simulink model "MSDRPrimaryLoop"  (R2021b)
settings: Solver=VariableStepAuto  StartTime=0.0  StopTime=250000  MaxStep=1  MinStep=0.01  RelTol=1e-3
undefined symbols (not defined in the file): a_f, A_free_PHX, a_g, A_h_PHX, beta, beta_t, bubbleGeneratorArea, bubbleGeneratorDh, bubbleGeneratorElevation, bubbleGeneratorLength, bubbleGeneratorVolume, bubbleSaturationLevel, bubbleSeparatorArea, bubbleSeparatorDiameter, bubbleSeparatorDo, bubbleSeparatorLength, bubbleSeparatorSlope, bypassRatio, C0, coreFlowArea, coreFuelVolume, coreLowerPlenumArea, coreLowerPlenumHydraulicDiameter, coreLowerPlenumLength, coreLowerPlenumVolume, coreUpperPlenumArea, coreUpperPlenumHydraulicDiameter, coreUpperPlenumLength, coreUpperPlenumVolume, coreVolume, cpGraphite, dissolusionRatio, dMin, dScale, dsmConst, DXeG, Fiss_factor, fuelChannelHydrualicDiameter, fuelChannelLength, fuelDepositRatio, fuelFraction, fuelGraphiteArea, fuelGraphiteHeatTransferCoefficient, gamma0, gamma1, gamma2, generatorDsm, graphiteKDiff, graphiteUnitCellThickness, initialIodineConcentration, InitialXeMolarConcentration, InjectionRatio, injectionRatio, iodineDecayConstant, IodineDecayConstant, iodineYield, kGraphite, kScale, Lam, lam ... (+59)
libraries: fl_lib x272, nesl_utility x105, SimscapeFluids_lib x24, slpidlib x1
(part 2 of 12)

== system MSDRPrimaryLoop/Chemical Processing/Bubble Generator ==
  XeIn : Inport
  GasIn : Inport  Port=2
  Add : Sum  Inputs=|++
  Delay One Step : Delay  DelayLength=1
  Gain : Gain  Gain=0.5
  GasCalc : Subsystem  mask{Volume=bubbleGeneratorVolume, VoidFraction=targetGeneratorVoidFraction}
      mask prompts: VoidFraction "TargetVoidFraction"
      settings: PortSchema="{\"entries\":[{\"content\":{\"sides\":[{\"content\":{\"connectorIds\":[\"In1\"]},\"type\":\"ConnectorPlacement.EquallySpacedRectSide\",\"uuid\":\"a8e1ce06-71c9-462d-8d5c-7a3e078b5544\"},{\"content\":{\"connectorIds\":[\"Out1\"],\"side\":\"RIGHT\"},\"type\":\"ConnectorPlacement.EquallySpacedRectSide\",\"uuid\":\"2c63a1ce-15e2-4b17-a432-f9f40781bd58\"},{\"content\":{\"connectorIds\":[\"LConn1\",\"LConn2\",\"LConn3\"],\"side\":\"TOP\"},\"type\":\"ConnectorPlacement.EquallySpacedRectSide\",\"uuid\":\"abc20e07-15eb-475f-be7f-cc96378523a1\"},{\"content\":{\"connectorIds\":[],\"side\":\"BOTTOM\"},\"type\":\"ConnectorPlacement.EquallySpacedRectSide\",\"uuid\":\"ab58f362-f4c2-4e86-bda0-802426066295\"}]},\"type\":\"ConnectorPlacement.EquallySpacedConnector\",\"uuid\":\"b54d49a9-048b-4912-bf18-92a7ef5e8aff\"}],\"packageUris\":[\"http://schema.mathworks.com/mf0/Connector/R2020b\"],\"version\":\"1.0\"}"
  PLossFunc : Subsystem
      settings: PortSchema="{\"entries\":[{\"content\":{\"sides\":[{\"content\":{\"connectorIds\":[\"Out1\",\"LConn1\"]},\"type\":\"ConnectorPlacement.EquallySpacedRectSide\",\"uuid\":\"95ca4545-c473-4e31-844b-c43557042c16\"},{\"content\":{\"connectorIds\":[\"RConn1\"],\"side\":\"RIGHT\"},\"type\":\"ConnectorPlacement.EquallySpacedRectSide\",\"uuid\":\"f9304c30-8684-4a05-a34b-3121610e628d\"},{\"content\":{\"connectorIds\":[],\"side\":\"TOP\"},\"type\":\"ConnectorPlacement.EquallySpacedRectSide\",\"uuid\":\"64c7a4d8-8539-4303-ae81-4015bd1451af\"}]},\"type\":\"ConnectorPlacement.EquallySpacedConnector\",\"uuid\":\"40c12b2f-fb9d-4a19-b6f1-e93ae1fd4d68\"}],\"packageUris\":[\"http://schema.mathworks.com/mf0/Connector/R2020b\"],\"version\":\"1.0\"}"
  Subsystem : Subsystem  mask{Volume=bubbleGeneratorArea*bubbleGeneratorLength, Area=bubbleGeneratorArea, Length=bubbleGeneratorLength, Dh=bubbleGeneratorDh, Elevation=bubbleGeneratorElevation, MinimumArea=bubbleGeneratorArea*0.5}
      mask prompts: Dh "Hydraulic Diameter"; MinimumArea "VenturiMinimumArea"
      settings: PortSchema="{\"entries\":[{\"content\":{\"sides\":[{\"content\":{\"connectorIds\":[\"LConn1\",\"In1\"]},\"type\":\"ConnectorPlacement.EquallySpacedRectSide\",\"uuid\":\"0f255306-ec83-4423-ac41-a2708bd1ec44\"},{\"content\":{\"connectorIds\":[\"RConn1\"],\"side\":\"RIGHT\"},\"type\":\"ConnectorPlacement.EquallySpacedRectSide\",\"uuid\":\"650fb4ea-7b32-4c45-8538-9785d9ca64bf\"},{\"content\":{\"connectorIds\":[],\"side\":\"TOP\"},\"type\":\"ConnectorPlacement.EquallySpacedRectSide\",\"uuid\":\"434d3568-54a4-4787-a287-69f15ef478cb\"},{\"content\":{\"connectorIds\":[\"RConn2\"],\"side\":\"BOTTOM\"},\"type\":\"ConnectorPlacement.EquallySpacedRectSide\",\"uuid\":\"5b0b510d-1175-4508-bbe9-65b563e28484\"}]},\"type\":\"ConnectorPlacement.EquallySpacedConnector\",\"uuid\":\"b18d9c84-3d71-444b-a89d-79c3dc70d4d9\"}],\"packageUris\":[\"http://schema.mathworks.com/mf0/Connector/R2020b\"],\"version\":\"1.0\"}"
  XenonCalc : Subsystem  mask{Volume=bubbleGeneratorVolume, Area=bubbleGeneratorArea, Length=bubbleGeneratorLength, Dh=bubbleGeneratorDh, Elevation=bubbleGeneratorElevation, Dsm=generatorDsm}
      mask prompts: Dh "Hydraulic Diameter"; Dsm "InjectedBubbleDiameter"
      settings: PortSchema="{\"entries\":[{\"content\":{\"sides\":[{\"content\":{\"connectorIds\":[\"LConn1\",\"In1\"]},\"type\":\"ConnectorPlacement.EquallySpacedRectSide\",\"uuid\":\"82f8e7e7-fd89-4597-952e-64db268d0190\"},{\"content\":{\"connectorIds\":[\"RConn1\",\"Out1\"],\"side\":\"RIGHT\"},\"type\":\"ConnectorPlacement.EquallySpacedRectSide\",\"uuid\":\"4b3edad1-18f8-43fa-96ee-a24bb3384b59\"},{\"content\":{\"connectorIds\":[\"In2\"],\"side\":\"TOP\"},\"type\":\"ConnectorPlacement.EquallySpacedRectSide\",\"uuid\":\"43d4f51d-f841-40d6-804e-7f238a90dabe\"},{\"content\":{\"connectorIds\":[\"In3\"],\"side\":\"BOTTOM\"},\"type\":\"ConnectorPlacement.EquallySpacedRectSide\",\"uuid\":\"350f2274-4108-4e6e-a637-0ae7118de3f0\"}]},\"type\":\"ConnectorPlacement.EquallySpacedConnector\",\"uuid\":\"d7e795ea-9d5d-4a8c-83ab-dab42197cc2f\"}],\"packageUris\":[\"http://schema.mathworks.com/mf0/Connector/R2020b\"],\"version\":\"1.0\"}"
  Inlet : PMIOPort  Side=Left
  Outlet : PMIOPort  Port=2  Side=Right
  XeOut : Outport
  GasOut : Outport  Port=2
  wires:
  XenonCalc/1(XeOut) -> XeOut/1
  Add/1 -> Gain/1
  GasCalc/1(GasOut) -> GasOut/1, Add/2
  Gain/1 -> Delay One Step/1
  GasIn/1 -> GasCalc/1(GasIn), Add/1
  Delay One Step/1 -> XenonCalc/3(GasRef), Subsystem/1(GasInRef)
  XeIn/1 -> XenonCalc/1(XeIn)
  PLossFunc/1(PLoss) -> XenonCalc/2(PLoss)
  connections:
  GasCalc/LConn1 -- XenonCalc/LConn1 -- Inlet/RConn1
  GasCalc/LConn3 -- PLossFunc/RConn1 -- Outlet/RConn1 -- Subsystem/RConn1
  GasCalc/LConn2 -- Subsystem/RConn2
  PLossFunc/LConn1 -- XenonCalc/RConn1 -- Subsystem/LConn1

== system MSDRPrimaryLoop/Chemical Processing/Bubble Separator ==
  XeIn : Inport  OutDataTypeStr=double  Unit=kg/s
  GasIn : Inport  Port=2
  Constant : Constant
  Demux : Demux  Outputs=2
  Mux : Mux  Inputs=2
  PS Abs : fl_lib/Physical Signals/Nonlinear Operators/PS Abs
      settings: SourceProductBaseCode=SS  InternalSimscapePortConfiguration="{\"Bottom\":[],\"Left\":[{\"id\":\"I\",\"label\":\"\",\"type\":\"input\"}],\"Right\":[{\"id\":\"O\",\"label\":\"\",\"type\":\"output\"}],\"Top\":[]}"
  PS-Simulink Converter : nesl_utility/PS-Simulink Converter  PhysicalDomain=network_engine_domain  SubClassName=ps_output  LeftPortType=input  RightPortType=output  PseudoPeriodic=off  Frequencies=[]  Unit=inherit  AffineConversion=off
      settings: SourceProductBaseCode=PW,SS
  Pipe (TL) : SimscapeFluids_lib/Thermal Liquid/Pipes & Fittings/Pipe (TL)  dynamic_compressibility=simscape.enum.onoff.on  inertia=simscape.enum.onoff.off  num_segments=1  pipe_length=bubbleSeparatorLength m  area=bubbleSeparatorArea m^2  Dh=bubbleSeparatorDiameter m  wall_spec=fluids.thermal_liquid.pipes_fittings.enum.wall_spec.rigid  Dh_rigid=bubbleSeparatorDiameter m  wall_compliance=1.2e-6 m/MPa  wall_time_constant=0.01 s  elevation_spec=foundation.enum.constant_variable.constant  elevation_gain=0 m  g=9.81 m/s^2  pressure_loss_spec=fluids.thermal_liquid.pipes_fittings.enum.PressureLossSpec.Haaland  length_add=1 m  roughness=15e-6 m  Re_friction_TLU=[400, 1000, 1500, 3000, 4000, 6000, 10000, 20000, 40000, 60000, 100000, 100000000]  friction_factor_TLU=[.264, .112, .071, .0417, .0387, .0268, .025, .0232, .0226, .022, .0214, .0214]  shape_factor=64  Re_lam=2000  Re_tur=4000  mdot_nominal=[.1, 1] kg/s  p_diff_nominal=[.001, .01] MPa  mdot_threshold=1e-6 kg/s  heat_transfer_spec=fluids.thermal_liquid.pipes_fittings.enum.HeatTransferSpec.Gnielinski  mdot_nominal_heat=[.1, 1] kg/s  T_in_nominal=[293.15, 293.15] K  T_out_nominal=[300, 300] K  p_in_nominal_heat=[.101325, .101325] MPa  T_wall_nominal=[303.15, 303.15] K  a_coeff=0.023  b_Re_power=0.8  c_Pr_power=0.4  Nu_lam=3.66  Re_Colburn_TLU=[100, 150, 1000]  Colburn_factor_TLU=[.019, .013, .002]  Re_Nu_TLU=[100, 150, 1000]  Pr_Nu_TLU=[1, 10]  Nu_TLU=[3.72, 4.21; 3.75, 4.44; 4.21, 7.15]  T0_vec=T0 K  p0_vec=P0 Pa  mdot0=0.1 kg/s
      settings: SourceProductBaseCode=SH
  Product : Product
  Subsystem : Subsystem
      settings: PortSchema="{\"entries\":[{\"content\":{\"sides\":[{\"content\":{\"connectorIds\":[\"In1\",\"In2\"]},\"type\":\"ConnectorPlacement.EquallySpacedRectSide\",\"uuid\":\"428c9e87-9ca6-4187-8542-12893d09804c\"},{\"content\":{\"connectorIds\":[\"Out1\"],\"side\":\"RIGHT\"},\"type\":\"ConnectorPlacement.EquallySpacedRectSide\",\"uuid\":\"49ffe6be-5da6-43ae-9c06-12a699a32540\"},{\"content\":{\"connectorIds\":[\"Out2\"],\"side\":\"TOP\"},\"type\":\"ConnectorPlacement.EquallySpacedRectSide\",\"uuid\":\"09f5b805-0e4a-4494-a05c-730d3143cb28\"},{\"content\":{\"connectorIds\":[\"RConn1\"],\"side\":\"BOTTOM\"},\"type\":\"ConnectorPlacement.EquallySpacedRectSide\",\"uuid\":\"f4e426df-1694-4b1d-823a-475b1a6b135f\"}]},\"type\":\"ConnectorPlacement.EquallySpacedConnector\",\"uuid\":\"8fc0cfcf-d77b-45e0-be8a-b32970fc4d69\"}],\"packageUris\":[\"http://schema.mathworks.com/mf0/Connector/R2020b\"],\"version\":\"1.0\"}"
  Subtract : Sum  Inputs=+-
  To Workspace : ToWorkspace  VariableName=divertedFlowRate  SaveFormat=Timeseries  SampleTime=50
  To Workspace2 : ToWorkspace  VariableName=separatorEffList  SaveFormat=Timeseries  SampleTime=50
  Volumetric Flow Rate Sensor (TL) : fl_lib/Thermal Liquid/Sensors/Volumetric Flow Rate Sensor (TL)
      settings: SourceProductBaseCode=SS  InternalSimscapePortConfiguration="{\"Bottom\":[],\"Left\":[{\"id\":\"A\",\"label\":\"A\",\"type\":\"foundation.thermal_liquid.thermal_liquid\"}],\"Right\":[{\"id\":\"B\",\"label\":\"B\",\"type\":\"foundation.thermal_liquid.thermal_liquid\"},{\"id\":\"V\",\"label\":\"V\",\"type\":\"output\"}],\"Top\":[]}"
  Inlet : PMIOPort  Side=Left
  Outlet : PMIOPort  Port=2  Side=Right
  XeOut : Outport
  GasOut : Outport  Port=2
  wires:
  XeIn/1 -> Demux/1
  Mux/1 -> XeOut/1
  Demux/1 -> Mux/1
  GasIn/1 -> Subsystem/1(GasIn)
  Subsystem/1(GasOut) -> GasOut/1
  PS-Simulink Converter/1 -> To Workspace/1, Subsystem/2(volRate)
  Constant/1 -> Subtract/1
  Demux/2 -> Product/1
  Subtract/1 -> Product/2
  Product/1 -> Mux/2
  Subsystem/2(SepEff) -> To Workspace2/1, Subtract/2
  connections:
  Volumetric Flow Rate Sensor (TL)/RConn1 -- Subsystem/RConn1 -- Pipe (TL)/LConn1
  Volumetric Flow Rate Sensor (TL)/RConn2 -- PS Abs/LConn1
  PS-Simulink Converter/LConn1 -- PS Abs/RConn1
  Inlet/RConn1 -- Volumetric Flow Rate Sensor (TL)/LConn1
  Outlet/RConn1 -- Pipe (TL)/RConn1

== system MSDRPrimaryLoop/Chemical Processing/ElevationPipe ==
  XeIn : Inport
  GasIn : Inport  Port=2
  Add : Sum  Inputs=|++
  Delay One Step : Delay  DelayLength=1
  Gain : Gain  Gain=0.5
  GasCalc : Subsystem  mask{Volume=Volume}
      settings: PortSchema="{\"entries\":[{\"content\":{\"sides\":[{\"content\":{\"connectorIds\":[\"In1\"]},\"type\":\"ConnectorPlacement.EquallySpacedRectSide\",\"uuid\":\"a8e1ce06-71c9-462d-8d5c-7a3e078b5544\"},{\"content\":{\"connectorIds\":[\"Out1\"],\"side\":\"RIGHT\"},\"type\":\"ConnectorPlacement.EquallySpacedRectSide\",\"uuid\":\"2c63a1ce-15e2-4b17-a432-f9f40781bd58\"},{\"content\":{\"connectorIds\":[\"LConn1\",\"LConn2\",\"LConn3\"],\"side\":\"TOP\"},\"type\":\"ConnectorPlacement.EquallySpacedRectSide\",\"uuid\":\"abc20e07-15eb-475f-be7f-cc96378523a1\"},{\"content\":{\"connectorIds\":[],\"side\":\"BOTTOM\"},\"type\":\"ConnectorPlacement.EquallySpacedRectSide\",\"uuid\":\"ab58f362-f4c2-4e86-bda0-802426066295\"}]},\"type\":\"ConnectorPlacement.EquallySpacedConnector\",\"uuid\":\"b54d49a9-048b-4912-bf18-92a7ef5e8aff\"}],\"packageUris\":[\"http://schema.mathworks.com/mf0/Connector/R2020b\"],\"version\":\"1.0\"}"
  PLossFunc : Subsystem
      settings: PortSchema="{\"entries\":[{\"content\":{\"sides\":[{\"content\":{\"connectorIds\":[\"Out1\",\"LConn1\"]},\"type\":\"ConnectorPlacement.EquallySpacedRectSide\",\"uuid\":\"95ca4545-c473-4e31-844b-c43557042c16\"},{\"content\":{\"connectorIds\":[\"RConn1\"],\"side\":\"RIGHT\"},\"type\":\"ConnectorPlacement.EquallySpacedRectSide\",\"uuid\":\"f9304c30-8684-4a05-a34b-3121610e628d\"},{\"content\":{\"connectorIds\":[],\"side\":\"TOP\"},\"type\":\"ConnectorPlacement.EquallySpacedRectSide\",\"uuid\":\"64c7a4d8-8539-4303-ae81-4015bd1451af\"}]},\"type\":\"ConnectorPlacement.EquallySpacedConnector\",\"uuid\":\"40c12b2f-fb9d-4a19-b6f1-e93ae1fd4d68\"}],\"packageUris\":[\"http://schema.mathworks.com/mf0/Connector/R2020b\"],\"version\":\"1.0\"}"
  Subsystem : Subsystem  mask{Volume=Volume, Area=Area, Length=Length, Dh=Dh, Elevation=Elevation}
      mask prompts: Dh "Hydraulic Diameter"
      settings: PortSchema="{\"entries\":[{\"content\":{\"sides\":[{\"content\":{\"connectorIds\":[\"LConn1\",\"In1\"]},\"type\":\"ConnectorPlacement.EquallySpacedRectSide\",\"uuid\":\"0f255306-ec83-4423-ac41-a2708bd1ec44\"},{\"content\":{\"connectorIds\":[\"RConn1\"],\"side\":\"RIGHT\"},\"type\":\"ConnectorPlacement.EquallySpacedRectSide\",\"uuid\":\"650fb4ea-7b32-4c45-8538-9785d9ca64bf\"},{\"content\":{\"connectorIds\":[],\"side\":\"TOP\"},\"type\":\"ConnectorPlacement.EquallySpacedRectSide\",\"uuid\":\"434d3568-54a4-4787-a287-69f15ef478cb\"},{\"content\":{\"connectorIds\":[\"RConn2\"],\"side\":\"BOTTOM\"},\"type\":\"ConnectorPlacement.EquallySpacedRectSide\",\"uuid\":\"5b0b510d-1175-4508-bbe9-65b563e28484\"}]},\"type\":\"ConnectorPlacement.EquallySpacedConnector\",\"uuid\":\"b18d9c84-3d71-444b-a89d-79c3dc70d4d9\"}],\"packageUris\":[\"http://schema.mathworks.com/mf0/Connector/R2020b\"],\"version\":\"1.0\"}"
  XenonCalc : Subsystem  mask{Volume=Volume, Area=Area, Length=Length, Dh=Dh, Elevation=Elevation}
      mask prompts: Dh "Hydraulic Diameter"
      settings: PortSchema="{\"entries\":[{\"content\":{\"sides\":[{\"content\":{\"connectorIds\":[\"LConn1\",\"In1\"]},\"type\":\"ConnectorPlacement.EquallySpacedRectSide\",\"uuid\":\"82f8e7e7-fd89-4597-952e-64db268d0190\"},{\"content\":{\"connectorIds\":[\"RConn1\",\"Out1\"],\"side\":\"RIGHT\"},\"type\":\"ConnectorPlacement.EquallySpacedRectSide\",\"uuid\":\"4b3edad1-18f8-43fa-96ee-a24bb3384b59\"},{\"content\":{\"connectorIds\":[\"In2\"],\"side\":\"TOP\"},\"type\":\"ConnectorPlacement.EquallySpacedRectSide\",\"uuid\":\"43d4f51d-f841-40d6-804e-7f238a90dabe\"},{\"content\":{\"connectorIds\":[\"In3\"],\"side\":\"BOTTOM\"},\"type\":\"ConnectorPlacement.EquallySpacedRectSide\",\"uuid\":\"350f2274-4108-4e6e-a637-0ae7118de3f0\"}]},\"type\":\"ConnectorPlacement.EquallySpacedConnector\",\"uuid\":\"d7e795ea-9d5d-4a8c-83ab-dab42197cc2f\"}],\"packageUris\":[\"http://schema.mathworks.com/mf0/Connector/R2020b\"],\"version\":\"1.0\"}"
  Inlet : PMIOPort  Side=Left
  Outlet : PMIOPort  Port=2  Side=Right
  XeOut : Outport
  GasOut : Outport  Port=2
  wires:
  XenonCalc/1(XeOut) -> XeOut/1
  Add/1 -> Gain/1
  GasCalc/1(GasOut) -> GasOut/1, Add/2
  Gain/1 -> Delay One Step/1
  GasIn/1 -> GasCalc/1(GasIn), Add/1
  Delay One Step/1 -> XenonCalc/3(GasRef), Subsystem/1(GasInRef)
  XeIn/1 -> XenonCalc/1(XeIn)
  PLossFunc/1(PLoss) -> XenonCalc/2(PLoss)
  connections:
  GasCalc/LConn1 -- XenonCalc/LConn1 -- Inlet/RConn1
  GasCalc/LConn3 -- PLossFunc/RConn1 -- Outlet/RConn1 -- Subsystem/RConn1
  GasCalc/LConn2 -- Subsystem/RConn2
  PLossFunc/LConn1 -- XenonCalc/RConn1 -- Subsystem/LConn1

== system MSDRPrimaryLoop/Chemical Processing/PipeLine ==
  XeIn : Inport  OutDataTypeStr=double  Unit=kg/s
  GasIn : Inport  Port=2
  Add : Sum  Inputs=|++
  Delay One Step : Delay  DelayLength=1
  Gain : Gain  Gain=0.5
  GasCalc : Subsystem  mask{Volume=pipeLineVolume}
      settings: PortSchema="{\"entries\":[{\"content\":{\"sides\":[{\"content\":{\"connectorIds\":[\"In1\"]},\"type\":\"ConnectorPlacement.EquallySpacedRectSide\",\"uuid\":\"a8e1ce06-71c9-462d-8d5c-7a3e078b5544\"},{\"content\":{\"connectorIds\":[\"Out1\"],\"side\":\"RIGHT\"},\"type\":\"ConnectorPlacement.EquallySpacedRectSide\",\"uuid\":\"2c63a1ce-15e2-4b17-a432-f9f40781bd58\"},{\"content\":{\"connectorIds\":[\"LConn1\",\"LConn2\",\"LConn3\"],\"side\":\"TOP\"},\"type\":\"ConnectorPlacement.EquallySpacedRectSide\",\"uuid\":\"abc20e07-15eb-475f-be7f-cc96378523a1\"},{\"content\":{\"connectorIds\":[],\"side\":\"BOTTOM\"},\"type\":\"ConnectorPlacement.EquallySpacedRectSide\",\"uuid\":\"ab58f362-f4c2-4e86-bda0-802426066295\"}]},\"type\":\"ConnectorPlacement.EquallySpacedConnector\",\"uuid\":\"b54d49a9-048b-4912-bf18-92a7ef5e8aff\"}],\"packageUris\":[\"http://schema.mathworks.com/mf0/Connector/R2020b\"],\"version\":\"1.0\"}"
  PLossFunc : Subsystem
      settings: PortSchema="{\"entries\":[{\"content\":{\"sides\":[{\"content\":{\"connectorIds\":[\"Out1\",\"LConn1\"]},\"type\":\"ConnectorPlacement.EquallySpacedRectSide\",\"uuid\":\"95ca4545-c473-4e31-844b-c43557042c16\"},{\"content\":{\"connectorIds\":[\"RConn1\"],\"side\":\"RIGHT\"},\"type\":\"ConnectorPlacement.EquallySpacedRectSide\",\"uuid\":\"f9304c30-8684-4a05-a34b-3121610e628d\"},{\"content\":{\"connectorIds\":[],\"side\":\"TOP\"},\"type\":\"ConnectorPlacement.EquallySpacedRectSide\",\"uuid\":\"64c7a4d8-8539-4303-ae81-4015bd1451af\"}]},\"type\":\"ConnectorPlacement.EquallySpacedConnector\",\"uuid\":\"40c12b2f-fb9d-4a19-b6f1-e93ae1fd4d68\"}],\"packageUris\":[\"http://schema.mathworks.com/mf0/Connector/R2020b\"],\"version\":\"1.0\"}"
  Subsystem : Subsystem  mask{Volume=pipeLineVolume, Area=pipeLineArea, Length=pipeLineLength, Dh=pipeLineDh, Elevation=pipeLineElevation, KLoss=pipeLineKLoss}
      mask prompts: Dh "Hydraulic Diameter"; KLoss "TotalKLoss"
      settings: PortSchema="{\"entries\":[{\"content\":{\"sides\":[{\"content\":{\"connectorIds\":[\"LConn1\",\"In1\"]},\"type\":\"ConnectorPlacement.EquallySpacedRectSide\",\"uuid\":\"0f255306-ec83-4423-ac41-a2708bd1ec44\"},{\"content\":{\"connectorIds\":[\"RConn1\"],\"side\":\"RIGHT\"},\"type\":\"ConnectorPlacement.EquallySpacedRectSide\",\"uuid\":\"650fb4ea-7b32-4c45-8538-9785d9ca64bf\"},{\"content\":{\"connectorIds\":[],\"side\":\"TOP\"},\"type\":\"ConnectorPlacement.EquallySpacedRectSide\",\"uuid\":\"434d3568-54a4-4787-a287-69f15ef478cb\"},{\"content\":{\"connectorIds\":[\"RConn2\"],\"side\":\"BOTTOM\"},\"type\":\"ConnectorPlacement.EquallySpacedRectSide\",\"uuid\":\"5b0b510d-1175-4508-bbe9-65b563e28484\"}]},\"type\":\"ConnectorPlacement.EquallySpacedConnector\",\"uuid\":\"b18d9c84-3d71-444b-a89d-79c3dc70d4d9\"}],\"packageUris\":[\"http://schema.mathworks.com/mf0/Connector/R2020b\"],\"version\":\"1.0\"}"
  XenonCalc : Subsystem  mask{Volume=pipeLineVolume, Area=pipeLineArea, Length=pipeLineLength, Dh=pipeLineDh, Elevation=pipeLineElevation, Dsm=generatorDsm}
      mask prompts: Dh "Hydraulic Diameter"; Dsm "InjectedBubbleDiameter"
      settings: PortSchema="{\"entries\":[{\"content\":{\"sides\":[{\"content\":{\"connectorIds\":[\"LConn1\",\"In1\"]},\"type\":\"ConnectorPlacement.EquallySpacedRectSide\",\"uuid\":\"82f8e7e7-fd89-4597-952e-64db268d0190\"},{\"content\":{\"connectorIds\":[\"RConn1\",\"Out1\"],\"side\":\"RIGHT\"},\"type\":\"ConnectorPlacement.EquallySpacedRectSide\",\"uuid\":\"4b3edad1-18f8-43fa-96ee-a24bb3384b59\"},{\"content\":{\"connectorIds\":[\"In2\"],\"side\":\"TOP\"},\"type\":\"ConnectorPlacement.EquallySpacedRectSide\",\"uuid\":\"43d4f51d-f841-40d6-804e-7f238a90dabe\"},{\"content\":{\"connectorIds\":[\"In3\"],\"side\":\"BOTTOM\"},\"type\":\"ConnectorPlacement.EquallySpacedRectSide\",\"uuid\":\"350f2274-4108-4e6e-a637-0ae7118de3f0\"}]},\"type\":\"ConnectorPlacement.EquallySpacedConnector\",\"uuid\":\"d7e795ea-9d5d-4a8c-83ab-dab42197cc2f\"}],\"packageUris\":[\"http://schema.mathworks.com/mf0/Connector/R2020b\"],\"version\":\"1.0\"}"
  Inlet : PMIOPort  Side=Left
  Outlet : PMIOPort  Port=2  Side=Right
  XeOut : Outport
  GasOut : Outport  Port=2
  wires:
  PLossFunc/1(PLoss) -> XenonCalc/2(PLoss)
  XeIn/1 -> XenonCalc/1(XeIn)
  XenonCalc/1(XeOut) -> XeOut/1
  Gain/1 -> Delay One Step/1
  GasCalc/1(GasOut) -> GasOut/1, Add/2
  GasIn/1 -> GasCalc/1(GasIn), Add/1
  Add/1 -> Gain/1
  Delay One Step/1 -> XenonCalc/3(GasRef), Subsystem/1(GasInRef)
  connections:
  PLossFunc/RConn1 -- GasCalc/LConn3 -- Subsystem/RConn1 -- Outlet/RConn1
  GasCalc/LConn1 -- XenonCalc/LConn1 -- Inlet/RConn1
  XenonCalc/RConn1 -- Subsystem/LConn1 -- PLossFunc/LConn1
  GasCalc/LConn2 -- Subsystem/RConn2

== system MSDRPrimaryLoop/Chemical Processing/VariablePressureControl ==
  note: // This will be zero if not connected at both ends of the pump. Use physical connection first.
      | If no pump is used in the system, there has to be a pressure difference between the separator and the pump suction for the separator to work.
      | This could be think as a variable conection point on the primary loop. The Pressure drop here is summary of all the pressure loss after the varaible connection point.
  XeIn : Inport  OutDataTypeStr=double  Unit=kg/s
  GasIn : Inport  Port=2
  Flow Resistance (TL) : fl_lib/Thermal Liquid/Elements/Flow Resistance (TL)  delta_p_nominal=nominalSeparatorDP Pa  mdot_nominal=nominalSeparatorFlowRate*nominalFuelDensity kg/s  area=bubbleSeparatorArea m^2  laminar_fraction=1e-3
      settings: SourceProductBaseCode=SS
  GasExpansion : Subsystem  ReferencedSubsystem=GasExpansion
      settings: PortSchema="{\"entries\":[{\"content\":{\"sides\":[{\"content\":{\"connectorIds\":[\"LConn1\",\"In1\"]},\"type\":\"ConnectorPlacement.EquallySpacedRectSide\",\"uuid\":\"50c89675-cb8a-4964-af62-cb2014507b1d\"},{\"content\":{\"connectorIds\":[\"RConn1\",\"Out1\"],\"side\":\"RIGHT\"},\"type\":\"ConnectorPlacement.EquallySpacedRectSide\",\"uuid\":\"6b3adc78-0be5-4682-9da0-6fd41ffc4e71\"},{\"content\":{\"connectorIds\":[],\"side\":\"TOP\"},\"type\":\"ConnectorPlacement.EquallySpacedRectSide\",\"uuid\":\"5158b46f-a496-48e4-90d6-6c6dcc9e237b\"}]},\"type\":\"ConnectorPlacement.EquallySpacedConnector\",\"uuid\":\"7ff0188e-dc19-44a0-a8cf-bde33949414f\"}],\"packageUris\":[\"http://schema.mathworks.com/mf0/Connector/R2020b\"],\"version\":\"1.0\"}"
  Inlet : PMIOPort  Side=Left
  Outlet : PMIOPort  Port=2  Side=Right
  XeOut : Outport
  GasOut : Outport  Port=2
  wires:
  GasExpansion/1 -> GasOut/1
  GasIn/1 -> GasExpansion/1
  XeIn/1 -> XeOut/1
  connections:
  GasExpansion/RConn1 -- Outlet/RConn1 -- Flow Resistance (TL)/RConn1
  GasExpansion/LConn1 -- Inlet/RConn1 -- Flow Resistance (TL)/LConn1

== system MSDRPrimaryLoop/Converge/Mixing ==
  note: The gas stream can be easily handled with ratio of liquid phase.
  Xe1 : Inport
  Xe2 : Inport  Port=2
  Gas1 : Inport  Port=3
  Gas2 : Inport  Port=4
  Add : Sum
  Add1 : Sum
  PS-Simulink Converter : nesl_utility/PS-Simulink Converter  PhysicalDomain=network_engine_domain  SubClassName=ps_output  LeftPortType=input  RightPortType=output  PseudoPeriodic=off  Frequencies=[]  Unit=inherit  AffineConversion=off
      settings: SourceProductBaseCode=PW,SS
  PS-Simulink Converter1 : nesl_utility/PS-Simulink Converter  PhysicalDomain=network_engine_domain  SubClassName=ps_output  LeftPortType=input  RightPortType=output  PseudoPeriodic=off  Frequencies=[]  Unit=inherit  AffineConversion=off
      settings: SourceProductBaseCode=PW,SS
  Product : Product
  Product1 : Product
  Mix1 : PMIOPort  Side=Left
  Mix2 : PMIOPort  Port=2  Side=Left
  XeOut : Outport
  GasOut : Outport  Port=2
  wires:
  PS-Simulink Converter/1 -> Product1/2
  PS-Simulink Converter1/1 -> Product/2
  Gas2/1 -> Product/1
  Gas1/1 -> Product1/1
  Product1/1 -> Add/1
  Product/1 -> Add/2
  Add/1 -> GasOut/1
  Add1/1 -> XeOut/1
  Xe1/1 -> Add1/1
  Xe2/1 -> Add1/2
  connections:
  Mix1/RConn1 -- PS-Simulink Converter/LConn1
  Mix2/RConn1 -- PS-Simulink Converter1/LConn1

== system MSDRPrimaryLoop/Converge/PhysicalNetwork ==
  Mass & Energy Flow Rate Sensor (TL) : fl_lib/Thermal Liquid/Sensors/Mass & Energy Flow Rate Sensor (TL)
      settings: SourceProductBaseCode=SS  InternalSimscapePortConfiguration="{\"Bottom\":[],\"Left\":[{\"id\":\"A\",\"label\":\"A\",\"type\":\"foundation.thermal_liquid.thermal_liquid\"}],\"Right\":[{\"id\":\"B\",\"label\":\"B\",\"type\":\"foundation.thermal_liquid.thermal_liquid\"},{\"id\":\"M\",\"label\":\"M\",\"type\":\"output\"},{\"id\":\"PHI\",\"label\":\"Phi\",\"type\":\"output\"}],\"Top\":[]}"
  Mass & Energy Flow Rate Sensor (TL)1 : fl_lib/Thermal Liquid/Sensors/Mass & Energy Flow Rate Sensor (TL)
      settings: SourceProductBaseCode=SS  InternalSimscapePortConfiguration="{\"Bottom\":[],\"Left\":[{\"id\":\"A\",\"label\":\"A\",\"type\":\"foundation.thermal_liquid.thermal_liquid\"}],\"Right\":[{\"id\":\"B\",\"label\":\"B\",\"type\":\"foundation.thermal_liquid.thermal_liquid\"},{\"id\":\"M\",\"label\":\"M\",\"type\":\"output\"},{\"id\":\"PHI\",\"label\":\"Phi\",\"type\":\"output\"}],\"Top\":[]}"
  Mass & Energy Flow Rate Sensor (TL)2 : fl_lib/Thermal Liquid/Sensors/Mass & Energy Flow Rate Sensor (TL)
      settings: SourceProductBaseCode=SS  InternalSimscapePortConfiguration="{\"Bottom\":[],\"Left\":[{\"id\":\"A\",\"label\":\"A\",\"type\":\"foundation.thermal_liquid.thermal_liquid\"}],\"Right\":[{\"id\":\"B\",\"label\":\"B\",\"type\":\"foundation.thermal_liquid.thermal_liquid\"},{\"id\":\"M\",\"label\":\"M\",\"type\":\"output\"},{\"id\":\"PHI\",\"label\":\"Phi\",\"type\":\"output\"}],\"Top\":[]}"
  PS Abs : fl_lib/Physical Signals/Nonlinear Operators/PS Abs
      settings: SourceProductBaseCode=SS  InternalSimscapePortConfiguration="{\"Bottom\":[],\"Left\":[{\"id\":\"I\",\"label\":\"\",\"type\":\"input\"}],\"Right\":[{\"id\":\"O\",\"label\":\"\",\"type\":\"output\"}],\"Top\":[]}"
  PS Abs1 : fl_lib/Physical Signals/Nonlinear Operators/PS Abs
      settings: SourceProductBaseCode=SS  InternalSimscapePortConfiguration="{\"Bottom\":[],\"Left\":[{\"id\":\"I\",\"label\":\"\",\"type\":\"input\"}],\"Right\":[{\"id\":\"O\",\"label\":\"\",\"type\":\"output\"}],\"Top\":[]}"
  PS Abs2 : fl_lib/Physical Signals/Nonlinear Operators/PS Abs
      settings: SourceProductBaseCode=SS  InternalSimscapePortConfiguration="{\"Bottom\":[],\"Left\":[{\"id\":\"I\",\"label\":\"\",\"type\":\"input\"}],\"Right\":[{\"id\":\"O\",\"label\":\"\",\"type\":\"output\"}],\"Top\":[]}"
  PS Constant : fl_lib/Physical Signals/Sources/PS Constant  constant=1e-6 kg/s
  PS Divide : fl_lib/Physical Signals/Functions/PS Divide
      settings: SourceProductBaseCode=SS
  PS Divide1 : fl_lib/Physical Signals/Functions/PS Divide
      settings: SourceProductBaseCode=SS
  PS Max : fl_lib/Physical Signals/Nonlinear Operators/PS Max
      settings: SourceProductBaseCode=SS  InternalSimscapePortConfiguration="{\"Bottom\":[],\"Left\":[{\"id\":\"I1\",\"label\":\"\",\"type\":\"input\"},{\"id\":\"I2\",\"label\":\"\",\"type\":\"input\"}],\"Right\":[{\"id\":\"O\",\"label\":\"\",\"type\":\"output\"}],\"Top\":[]}"
  Subsystem : Subsystem
  MainIn : PMIOPort  Side=Left
  SideIn : PMIOPort  Port=2  Side=Left
  MainRatio : PMIOPort  Port=3  Side=Right
  SideRatio : PMIOPort  Port=4  Side=Right
  TotalOut : PMIOPort  Port=5  Side=Right
  connections:
  Subsystem/LConn1 -- Mass & Energy Flow Rate Sensor (TL)/RConn1
  Mass & Energy Flow Rate Sensor (TL)/RConn2 -- PS Abs/LConn1
  Mass & Energy Flow Rate Sensor (TL)/LConn1 -- MainIn/RConn1
  Subsystem/LConn2 -- Mass & Energy Flow Rate Sensor (TL)1/RConn1
  Mass & Energy Flow Rate Sensor (TL)1/RConn2 -- PS Abs1/LConn1
  Mass & Energy Flow Rate Sensor (TL)1/LConn1 -- SideIn/RConn1
  Subsystem/RConn1 -- Mass & Energy Flow Rate Sensor (TL)2/LConn1
  TotalOut/RConn1 -- Mass & Energy Flow Rate Sensor (TL)2/RConn1
  Mass & Energy Flow Rate Sensor (TL)2/RConn2 -- PS Abs2/LConn1
  PS Abs2/RConn1 -- PS Max/LConn1
  PS Max/LConn2 -- PS Constant/RConn1
  PS Abs1/RConn1 -- PS Divide/LConn1
  PS Max/RConn1 -- PS Divide1/LConn2 -- PS Divide/LConn2
  PS Divide/RConn1 -- SideRatio/RConn1
  PS Abs/RConn1 -- PS Divide1/LConn1
  PS Divide1/RConn1 -- MainRatio/RConn1

== system MSDRPrimaryLoop/Diverge/Subsystem1 ==
  note: Handle divide by zero.
  MainXeRate : fl_lib/Physical Signals/Functions/PS Divide
      settings: SourceProductBaseCode=SS
  Mass & Energy Flow Rate Sensor (TL) : fl_lib/Thermal Liquid/Sensors/Mass & Energy Flow Rate Sensor (TL)
      settings: SourceProductBaseCode=SS  InternalSimscapePortConfiguration="{\"Bottom\":[],\"Left\":[{\"id\":\"A\",\"label\":\"A\",\"type\":\"foundation.thermal_liquid.thermal_liquid\"}],\"Right\":[{\"id\":\"B\",\"label\":\"B\",\"type\":\"foundation.thermal_liquid.thermal_liquid\"},{\"id\":\"M\",\"label\":\"M\",\"type\":\"output\"},{\"id\":\"PHI\",\"label\":\"Phi\",\"type\":\"output\"}],\"Top\":[]}"
  Mass & Energy Flow Rate Sensor (TL)1 : fl_lib/Thermal Liquid/Sensors/Mass & Energy Flow Rate Sensor (TL)
      settings: SourceProductBaseCode=SS  InternalSimscapePortConfiguration="{\"Bottom\":[],\"Left\":[{\"id\":\"A\",\"label\":\"A\",\"type\":\"foundation.thermal_liquid.thermal_liquid\"}],\"Right\":[{\"id\":\"B\",\"label\":\"B\",\"type\":\"foundation.thermal_liquid.thermal_liquid\"},{\"id\":\"M\",\"label\":\"M\",\"type\":\"output\"},{\"id\":\"PHI\",\"label\":\"Phi\",\"type\":\"output\"}],\"Top\":[]}"
  Mass & Energy Flow Rate Sensor (TL)2 : fl_lib/Thermal Liquid/Sensors/Mass & Energy Flow Rate Sensor (TL)
      settings: SourceProductBaseCode=SS  InternalSimscapePortConfiguration="{\"Bottom\":[],\"Left\":[{\"id\":\"A\",\"label\":\"A\",\"type\":\"foundation.thermal_liquid.thermal_liquid\"}],\"Right\":[{\"id\":\"B\",\"label\":\"B\",\"type\":\"foundation.thermal_liquid.thermal_liquid\"},{\"id\":\"M\",\"label\":\"M\",\"type\":\"output\"},{\"id\":\"PHI\",\"label\":\"Phi\",\"type\":\"output\"}],\"Top\":[]}"
  PS Abs : fl_lib/Physical Signals/Nonlinear Operators/PS Abs
      settings: SourceProductBaseCode=SS  InternalSimscapePortConfiguration="{\"Bottom\":[],\"Left\":[{\"id\":\"I\",\"label\":\"\",\"type\":\"input\"}],\"Right\":[{\"id\":\"O\",\"label\":\"\",\"type\":\"output\"}],\"Top\":[]}"
  PS Abs1 : fl_lib/Physical Signals/Nonlinear Operators/PS Abs
      settings: SourceProductBaseCode=SS  InternalSimscapePortConfiguration="{\"Bottom\":[],\"Left\":[{\"id\":\"I\",\"label\":\"\",\"type\":\"input\"}],\"Right\":[{\"id\":\"O\",\"label\":\"\",\"type\":\"output\"}],\"Top\":[]}"
  PS Abs2 : fl_lib/Physical Signals/Nonlinear Operators/PS Abs
      settings: SourceProductBaseCode=SS  InternalSimscapePortConfiguration="{\"Bottom\":[],\"Left\":[{\"id\":\"I\",\"label\":\"\",\"type\":\"input\"}],\"Right\":[{\"id\":\"O\",\"label\":\"\",\"type\":\"output\"}],\"Top\":[]}"
  PS Constant : fl_lib/Physical Signals/Sources/PS Constant  constant=1e-6 kg/s
  PS Max : fl_lib/Physical Signals/Nonlinear Operators/PS Max
      settings: SourceProductBaseCode=SS  InternalSimscapePortConfiguration="{\"Bottom\":[],\"Left\":[{\"id\":\"I1\",\"label\":\"\",\"type\":\"input\"},{\"id\":\"I2\",\"label\":\"\",\"type\":\"input\"}],\"Right\":[{\"id\":\"O\",\"label\":\"\",\"type\":\"output\"}],\"Top\":[]}"
  PS-Simulink Converter : nesl_utility/PS-Simulink Converter  PhysicalDomain=network_engine_domain  SubClassName=ps_output  LeftPortType=input  RightPortType=output  PseudoPeriodic=off  Frequencies=[]  Unit=inherit  AffineConversion=off
      settings: SourceProductBaseCode=PW,SS
  PS-Simulink Converter2 : nesl_utility/PS-Simulink Converter  PhysicalDomain=network_engine_domain  SubClassName=ps_output  LeftPortType=input  RightPortType=output  PseudoPeriodic=off  Frequencies=[]  Unit=inherit  AffineConversion=off
      settings: SourceProductBaseCode=PW,SS
  SideXeRate : fl_lib/Physical Signals/Functions/PS Divide
      settings: SourceProductBaseCode=SS
  Subsystem : Subsystem
  Inlet : PMIOPort  Side=Left
  MainOut : PMIOPort  Port=2  Side=Right
  SideOut : PMIOPort  Port=3  Side=Right
  MainRatio : Outport
  SideRatio : Outport  Port=2
  wires:
  PS-Simulink Converter2/1 -> MainRatio/1
  PS-Simulink Converter/1 -> SideRatio/1
  connections:
  MainXeRate/LConn1 -- PS Abs2/RConn1
  Mass & Energy Flow Rate Sensor (TL)/RConn1 -- Subsystem/LConn1
  Mass & Energy Flow Rate Sensor (TL)1/RConn1 -- SideOut/RConn1
  Mass & Energy Flow Rate Sensor (TL)1/RConn2 -- PS Abs1/LConn1
  Mass & Energy Flow Rate Sensor (TL)1/LConn1 -- Subsystem/RConn2
  PS Abs/RConn1 -- PS Max/LConn1
  PS Constant/RConn1 -- PS Max/LConn2
  PS Abs1/RConn1 -- SideXeRate/LConn1
  MainXeRate/RConn1 -- PS-Simulink Converter2/LConn1
  PS Abs2/LConn1 -- Mass & Energy Flow Rate Sensor (TL)2/RConn2
  SideXeRate/RConn1 -- PS-Simulink Converter/LConn1
  PS Max/RConn1 -- MainXeRate/LConn2 -- SideXeRate/LConn2
  Mass & Energy Flow Rate Sensor (TL)/RConn2 -- PS Abs/LConn1
  Mass & Energy Flow Rate Sensor (TL)2/LConn1 -- Subsystem/RConn1
  Mass & Energy Flow Rate Sensor (TL)/LConn1 -- Inlet/RConn1
  Mass & Energy Flow Rate Sensor (TL)2/RConn1 -- MainOut/RConn1

== system MSDRPrimaryLoop/Ideal Expansion//Drain Tank/Coupled ==
  DrainTank : fl_lib/Thermal Liquid/Elements/Reservoir (TL)  pressure_spec=foundation.enum.pressure_spec.specified  reservoir_pressure=P0 Pa  reservoir_temperature=T0 K  area=0.01 m^2
      settings: SourceProductBaseCode=SS
  TotalIn : PMIOPort  Side=Left
  Inlet : PMIOPort  Port=2  Side=Right
  connections:
  Inlet/RConn1 -- TotalIn/RConn1 -- DrainTank/LConn1

== system MSDRPrimaryLoop/Ideal Expansion//Drain Tank/Segregate ==
  SimpleOverFlowTank : fl_lib/Thermal Liquid/Elements/Reservoir (TL)  pressure_spec=foundation.enum.pressure_spec.specified  reservoir_pressure=P0 Pa  reservoir_temperature=T0 K  area=0.01 m^2
      settings: SourceProductBaseCode=SS
  SimpleOverFlowTank1 : fl_lib/Thermal Liquid/Elements/Reservoir (TL)  pressure_spec=foundation.enum.pressure_spec.specified  reservoir_pressure=P0 Pa  reservoir_temperature=T0 K  area=0.01 m^2
      settings: SourceProductBaseCode=SS
  TotalIn : PMIOPort  Side=Left
  Inlet : PMIOPort  Port=2  Side=Right
  connections:
  SimpleOverFlowTank/LConn1 -- TotalIn/RConn1
  SimpleOverFlowTank1/LConn1 -- Inlet/RConn1

== system MSDRPrimaryLoop/PHX/PHX Ideal ==
  note: The outlet temperature of the PHX is controlled as a constant. The pressure drop is scaled with the square of the volume flowrate. This is primarily used for xenon calculation.
  XeIn : Inport
  GasIn : Inport  Port=2
  Add : Sum  Inputs=|++
  Delay One Step : Delay  DelayLength=1  InitialCondition=0.02
  Gain : Gain  Gain=0.5
  GasCalc : Subsystem  mask{PipeVolume=PHXVolume}
      mask prompts: PipeVolume "Volume"
      settings: PortSchema="{\"entries\":[{\"content\":{\"sides\":[{\"content\":{\"connectorIds\":[\"In1\"]},\"type\":\"ConnectorPlacement.EquallySpacedRectSide\",\"uuid\":\"a8e1ce06-71c9-462d-8d5c-7a3e078b5544\"},{\"content\":{\"connectorIds\":[\"Out1\"],\"side\":\"RIGHT\"},\"type\":\"ConnectorPlacement.EquallySpacedRectSide\",\"uuid\":\"2c63a1ce-15e2-4b17-a432-f9f40781bd58\"},{\"content\":{\"connectorIds\":[\"LConn1\",\"LConn2\",\"LConn3\"],\"side\":\"TOP\"},\"type\":\"ConnectorPlacement.EquallySpacedRectSide\",\"uuid\":\"abc20e07-15eb-475f-be7f-cc96378523a1\"},{\"content\":{\"connectorIds\":[],\"side\":\"BOTTOM\"},\"type\":\"ConnectorPlacement.EquallySpacedRectSide\",\"uuid\":\"ab58f362-f4c2-4e86-bda0-802426066295\"}]},\"type\":\"ConnectorPlacement.EquallySpacedConnector\",\"uuid\":\"b54d49a9-048b-4912-bf18-92a7ef5e8aff\"}],\"packageUris\":[\"http://schema.mathworks.com/mf0/Connector/R2020b\"],\"version\":\"1.0\"}"
  PHXIdeal : Subsystem
      settings: PortSchema="{\"entries\":[{\"content\":{\"sides\":[{\"content\":{\"connectorIds\":[\"LConn1\"]},\"type\":\"ConnectorPlacement.EquallySpacedRectSide\",\"uuid\":\"f66bece2-fdc4-4c5c-8b9b-b9978f494d53\"},{\"content\":{\"connectorIds\":[\"RConn1\"],\"side\":\"RIGHT\"},\"type\":\"ConnectorPlacement.EquallySpacedRectSide\",\"uuid\":\"48186cbd-a433-437a-a956-52e0dc00c30c\"},{\"content\":{\"connectorIds\":[],\"side\":\"TOP\"},\"type\":\"ConnectorPlacement.EquallySpacedRectSide\",\"uuid\":\"cd990d09-c0f9-4846-88b8-fe01d85fbb00\"},{\"content\":{\"connectorIds\":[\"RConn2\"],\"side\":\"BOTTOM\"},\"type\":\"ConnectorPlacement.EquallySpacedRectSide\",\"uuid\":\"c2d21c1c-5d2e-4128-be09-2d665ea38132\"}]},\"type\":\"ConnectorPlacement.EquallySpacedConnector\",\"uuid\":\"00e4a5dc-c184-4d43-a987-caabcada1902\"}],\"packageUris\":[\"http://schema.mathworks.com/mf0/Connector/R2020b\"],\"version\":\"1.0\"}"
  PS-Simulink Converter : nesl_utility/PS-Simulink Converter  PhysicalDomain=network_engine_domain  SubClassName=ps_output  LeftPortType=input  RightPortType=output  PseudoPeriodic=off  Frequencies=[]  Unit=inherit  AffineConversion=off
      settings: SourceProductBaseCode=PW,SS
  Pressure & Temperature Sensor (TL) : fl_lib/Thermal Liquid/Sensors/Pressure & Temperature Sensor (TL)
      settings: SourceProductBaseCode=SS  InternalSimscapePortConfiguration="{\"Bottom\":[],\"Left\":[{\"id\":\"A\",\"label\":\"A\",\"type\":\"foundation.thermal_liquid.thermal_liquid\"}],\"Right\":[{\"id\":\"B\",\"label\":\"B\",\"type\":\"foundation.thermal_liquid.thermal_liquid\"},{\"id\":\"P\",\"label\":\"P\",\"type\":\"output\"},{\"id\":\"T\",\"label\":\"T\",\"type\":\"output\"}],\"Top\":[]}"
  XenonCalc : Subsystem  mask{Volume=PHXVolume, Area=FlowArea, Length=PHXLength, Dh=PHXHydraulicDiameter, Elevation=0}
      mask prompts: Dh "Hydraulic Diameter"
      settings: PortSchema="{\"entries\":[{\"content\":{\"sides\":[{\"content\":{\"connectorIds\":[\"LConn1\",\"In1\"]},\"type\":\"ConnectorPlacement.EquallySpacedRectSide\",\"uuid\":\"82f8e7e7-fd89-4597-952e-64db268d0190\"},{\"content\":{\"connectorIds\":[\"RConn1\",\"Out1\"],\"side\":\"RIGHT\"},\"type\":\"ConnectorPlacement.EquallySpacedRectSide\",\"uuid\":\"4b3edad1-18f8-43fa-96ee-a24bb3384b59\"},{\"content\":{\"connectorIds\":[\"In2\"],\"side\":\"TOP\"},\"type\":\"ConnectorPlacement.EquallySpacedRectSide\",\"uuid\":\"43d4f51d-f841-40d6-804e-7f238a90dabe\"},{\"content\":{\"connectorIds\":[\"In3\"],\"side\":\"BOTTOM\"},\"type\":\"ConnectorPlacement.EquallySpacedRectSide\",\"uuid\":\"350f2274-4108-4e6e-a637-0ae7118de3f0\"}]},\"type\":\"ConnectorPlacement.EquallySpacedConnector\",\"uuid\":\"d7e795ea-9d5d-4a8c-83ab-dab42197cc2f\"}],\"packageUris\":[\"http://schema.mathworks.com/mf0/Connector/R2020b\"],\"version\":\"1.0\"}"
  Inlet : PMIOPort  Side=Left
  Outlet : PMIOPort  Port=2  Side=Right
  XeOut : Outport
  GasOut : Outport  Port=2
  wires:
  XenonCalc/1(XeOut) -> XeOut/1
  XeIn/1 -> XenonCalc/1(XeIn)
  Gain/1 -> Delay One Step/1
  Delay One Step/1 -> XenonCalc/3(GasRef)
  GasIn/1 -> GasCalc/1(GasIn), Add/1
  GasCalc/1(GasOut) -> GasOut/1, Add/2
  Add/1 -> Gain/1
  PS-Simulink Converter/1 -> XenonCalc/2(PLoss)
  connections:
  GasCalc/LConn2 -- PHXIdeal/RConn2
  PHXIdeal/RConn1 -- Pressure & Temperature Sensor (TL)/RConn1 -- Outlet/RConn1 -- GasCalc/LConn3
  PHXIdeal/LConn1 -- Pressure & Temperature Sensor (TL)/LConn1 -- XenonCalc/RConn1 -- GasCalc/LConn1
  XenonCalc/LConn1 -- Inlet/RConn1
  PS-Simulink Converter/LConn1 -- Pressure & Temperature Sensor (TL)/RConn2

== system MSDRPrimaryLoop/PHX/PHX Physical ==
  XeIn : Inport
  GasIn : Inport  Port=2
  Add : Sum  Inputs=|++
  Delay One Step : Delay  DelayLength=1
  Gain : Gain  Gain=0.5
  GasCalc1 : Subsystem  mask{PipeVolume=PHXVolume}
      mask prompts: PipeVolume "Volume"
      settings: PortSchema="{\"entries\":[{\"content\":{\"sides\":[{\"content\":{\"connectorIds\":[\"In1\"]},\"type\":\"ConnectorPlacement.EquallySpacedRectSide\",\"uuid\":\"a8e1ce06-71c9-462d-8d5c-7a3e078b5544\"},{\"content\":{\"connectorIds\":[\"Out1\"],\"side\":\"RIGHT\"},\"type\":\"ConnectorPlacement.EquallySpacedRectSide\",\"uuid\":\"2c63a1ce-15e2-4b17-a432-f9f40781bd58\"},{\"content\":{\"connectorIds\":[\"LConn1\",\"LConn2\",\"LConn3\"],\"side\":\"TOP\"},\"type\":\"ConnectorPlacement.EquallySpacedRectSide\",\"uuid\":\"abc20e07-15eb-475f-be7f-cc96378523a1\"},{\"content\":{\"connectorIds\":[],\"side\":\"BOTTOM\"},\"type\":\"ConnectorPlacement.EquallySpacedRectSide\",\"uuid\":\"ab58f362-f4c2-4e86-bda0-802426066295\"}]},\"type\":\"ConnectorPlacement.EquallySpacedConnector\",\"uuid\":\"b54d49a9-048b-4912-bf18-92a7ef5e8aff\"}],\"packageUris\":[\"http://schema.mathworks.com/mf0/Connector/R2020b\"],\"version\":\"1.0\"}"
  PHXPhysics : Subsystem
      settings: PortSchema="{\"entries\":[{\"content\":{\"sides\":[{\"content\":{\"connectorIds\":[\"LConn1\",\"In1\"]},\"type\":\"ConnectorPlacement.EquallySpacedRectSide\",\"uuid\":\"f66bece2-fdc4-4c5c-8b9b-b9978f494d53\"},{\"content\":{\"connectorIds\":[\"RConn1\"],\"side\":\"RIGHT\"},\"type\":\"ConnectorPlacement.EquallySpacedRectSide\",\"uuid\":\"48186cbd-a433-437a-a956-52e0dc00c30c\"},{\"content\":{\"connectorIds\":[],\"side\":\"TOP\"},\"type\":\"ConnectorPlacement.EquallySpacedRectSide\",\"uuid\":\"cd990d09-c0f9-4846-88b8-fe01d85fbb00\"},{\"content\":{\"connectorIds\":[\"RConn2\"],\"side\":\"BOTTOM\"},\"type\":\"ConnectorPlacement.EquallySpacedRectSide\",\"uuid\":\"c2d21c1c-5d2e-4128-be09-2d665ea38132\"}]},\"type\":\"ConnectorPlacement.EquallySpacedConnector\",\"uuid\":\"00e4a5dc-c184-4d43-a987-caabcada1902\"}],\"packageUris\":[\"http://schema.mathworks.com/mf0/Connector/R2020b\"],\"version\":\"1.0\"}"
  XenonCalc1 : Subsystem  mask{PipeVolume=PHXVolume, PipeArea=FlowArea, PipeLength=ChannelLength, Dh=Dh}
      mask prompts: PipeVolume "Volume"; PipeArea "Area"; PipeLength "Length"; Dh "Hydraulic Diameter"
      settings: PortSchema="{\"entries\":[{\"content\":{\"sides\":[{\"content\":{\"connectorIds\":[\"LConn1\",\"In1\"]},\"type\":\"ConnectorPlacement.EquallySpacedRectSide\",\"uuid\":\"82f8e7e7-fd89-4597-952e-64db268d0190\"},{\"content\":{\"connectorIds\":[\"RConn1\",\"Out1\"],\"side\":\"RIGHT\"},\"type\":\"ConnectorPlacement.EquallySpacedRectSide\",\"uuid\":\"4b3edad1-18f8-43fa-96ee-a24bb3384b59\"},{\"content\":{\"connectorIds\":[],\"side\":\"TOP\"},\"type\":\"ConnectorPlacement.EquallySpacedRectSide\",\"uuid\":\"43d4f51d-f841-40d6-804e-7f238a90dabe\"},{\"content\":{\"connectorIds\":[\"In2\"],\"side\":\"BOTTOM\"},\"type\":\"ConnectorPlacement.EquallySpacedRectSide\",\"uuid\":\"350f2274-4108-4e6e-a637-0ae7118de3f0\"}]},\"type\":\"ConnectorPlacement.EquallySpacedConnector\",\"uuid\":\"d7e795ea-9d5d-4a8c-83ab-dab42197cc2f\"}],\"packageUris\":[\"http://schema.mathworks.com/mf0/Connector/R2020b\"],\"version\":\"1.0\"}"
  Inlet : PMIOPort  Side=Left
  Outlet : PMIOPort  Port=2  Side=Right
  XeOut : Outport
  GasOut : Outport  Port=2
  wires:
  XenonCalc1/1(XeOut) -> XeOut/1
  XeIn/1 -> XenonCalc1/1(XeIn)
  Gain/1 -> Delay One Step/1
  Delay One Step/1 -> XenonCalc1/2(GasRef), PHXPhysics/1(GasInRef)
  GasIn/1 -> GasCalc1/1(GasIn), Add/1
  GasCalc1/1(GasOut) -> GasOut/1, Add/2
  Add/1 -> Gain/1
  connections:
  GasCalc1/LConn2 -- PHXPhysics/RConn2
  PHXPhysics/RConn1 -- Outlet/RConn1 -- GasCalc1/LConn3
  PHXPhysics/LConn1 -- GasCalc1/LConn1 -- XenonCalc1/RConn1
  XenonCalc1/LConn1 -- Inlet/RConn1

== system MSDRPrimaryLoop/Pump/PumpIdeal ==
  XeIn : Inport
  GasIn : Inport  Port=2
  Add : Sum  Inputs=|++
  Delay One Step : Delay  DelayLength=1
  Gain : Gain  Gain=0.5
  GasCalcRegular : Subsystem  VariantControl=NoRemoval  mask{PipeVolume=PumpVolume}
      mask prompts: PipeVolume "Volume"
      settings: PortSchema="{\"entries\":[{\"content\":{\"sides\":[{\"content\":{\"connectorIds\":[\"In1\"]},\"type\":\"ConnectorPlacement.EquallySpacedRectSide\",\"uuid\":\"a8e1ce06-71c9-462d-8d5c-7a3e078b5544\"},{\"content\":{\"connectorIds\":[\"Out1\"],\"side\":\"RIGHT\"},\"type\":\"ConnectorPlacement.EquallySpacedRectSide\",\"uuid\":\"2c63a1ce-15e2-4b17-a432-f9f40781bd58\"},{\"content\":{\"connectorIds\":[\"LConn1\",\"LConn2\",\"LConn3\"],\"side\":\"TOP\"},\"type\":\"ConnectorPlacement.EquallySpacedRectSide\",\"uuid\":\"abc20e07-15eb-475f-be7f-cc96378523a1\"},{\"content\":{\"connectorIds\":[],\"side\":\"BOTTOM\"},\"type\":\"ConnectorPlacement.EquallySpacedRectSide\",\"uuid\":\"ab58f362-f4c2-4e86-bda0-802426066295\"}]},\"type\":\"ConnectorPlacement.EquallySpacedConnector\",\"uuid\":\"b54d49a9-048b-4912-bf18-92a7ef5e8aff\"}],\"packageUris\":[\"http://schema.mathworks.com/mf0/Connector/R2020b\"],\"version\":\"1.0\"}"
  Ideal Flowrate Pump : Subsystem
      settings: PortSchema="{\"entries\":[{\"content\":{\"sides\":[{\"content\":{\"connectorIds\":[\"LConn1\"]},\"type\":\"ConnectorPlacement.EquallySpacedRectSide\",\"uuid\":\"dfa2aa95-b0f6-4d42-b52c-ac64f68b4332\"},{\"content\":{\"connectorIds\":[\"RConn1\"],\"side\":\"RIGHT\"},\"type\":\"ConnectorPlacement.EquallySpacedRectSide\",\"uuid\":\"4e233f45-275b-4a62-b54f-a26261252d76\"},{\"content\":{\"connectorIds\":[],\"side\":\"TOP\"},\"type\":\"ConnectorPlacement.EquallySpacedRectSide\",\"uuid\":\"4d56cee6-54c9-4b53-b595-9dd9843d1812\"},{\"content\":{\"connectorIds\":[\"RConn2\"],\"side\":\"BOTTOM\"},\"type\":\"ConnectorPlacement.EquallySpacedRectSide\",\"uuid\":\"5b59abd0-5c01-4c9b-8b33-a5a665899d43\"}]},\"type\":\"ConnectorPlacement.EquallySpacedConnector\",\"uuid\":\"08118153-6206-4ac8-9187-5e3d4b128de1\"}],\"packageUris\":[\"http://schema.mathworks.com/mf0/Connector/R2020b\"],\"version\":\"1.0\"}"
  XenonCalcPump : Subsystem  mask{PipeVolume=PumpVolume, dsm=0.001*dScale, km=0.0005*kScale}
      mask prompts: PipeVolume "Volume"; dsm "Sauter Mean Diameter"; km "Mass Transfer Coefficient"
      settings: PortSchema="{\"entries\":[{\"content\":{\"sides\":[{\"content\":{\"connectorIds\":[\"LConn1\",\"In1\"]},\"type\":\"ConnectorPlacement.EquallySpacedRectSide\",\"uuid\":\"82f8e7e7-fd89-4597-952e-64db268d0190\"},{\"content\":{\"connectorIds\":[\"RConn1\",\"Out1\"],\"side\":\"RIGHT\"},\"type\":\"ConnectorPlacement.EquallySpacedRectSide\",\"uuid\":\"4b3edad1-18f8-43fa-96ee-a24bb3384b59\"},{\"content\":{\"connectorIds\":[],\"side\":\"TOP\"},\"type\":\"ConnectorPlacement.EquallySpacedRectSide\",\"uuid\":\"43d4f51d-f841-40d6-804e-7f238a90dabe\"},{\"content\":{\"connectorIds\":[\"In2\"],\"side\":\"BOTTOM\"},\"type\":\"ConnectorPlacement.EquallySpacedRectSide\",\"uuid\":\"350f2274-4108-4e6e-a637-0ae7118de3f0\"}]},\"type\":\"ConnectorPlacement.EquallySpacedConnector\",\"uuid\":\"d7e795ea-9d5d-4a8c-83ab-dab42197cc2f\"}],\"packageUris\":[\"http://schema.mathworks.com/mf0/Connector/R2020b\"],\"version\":\"1.0\"}"
  Inlet : PMIOPort  Side=Left
  Outlet : PMIOPort  Port=2  Side=Right
  XeOut : Outport
  GasOut : Outport  Port=2
  wires:
  GasIn/1 -> GasCalcRegular/1(GasIn), Add/1
  Add/1 -> Gain/1
  Gain/1 -> Delay One Step/1
  GasCalcRegular/1(GasOut) -> GasOut/1, Add/2
  XeIn/1 -> XenonCalcPump/1(XeIn)
  Delay One Step/1 -> XenonCalcPump/2(GasRef)
  XenonCalcPump/1(XeOut) -> XeOut/1
  connections:
  Ideal Flowrate Pump/RConn1 -- GasCalcRegular/LConn3 -- Outlet/RConn1
  GasCalcRegular/LConn2 -- Ideal Flowrate Pump/RConn2
  GasCalcRegular/LConn1 -- XenonCalcPump/LConn1 -- Inlet/RConn1
  XenonCalcPump/RConn1 -- Ideal Flowrate Pump/LConn1
